simulink model "DFexample"  (R2017a)
settings: Solver=FixedStepAuto  StartTime=0.0  StopTime=600  FixedStep=0.01  RelTol=1e-3
settings Model: Creator=bhannigan  LastModifiedBy=bhannigan

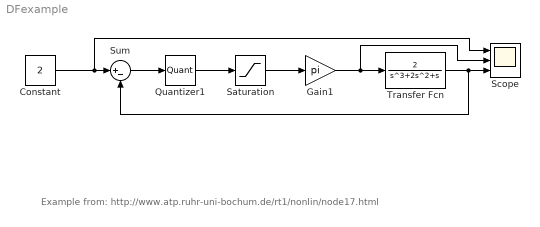
== system DFexample ==
  note: Example from: http://www.atp.ruhr-uni-bochum.de/rt1/nonlin/node17.html
  Constant : Constant  Value=2
  Gain1 : Gain  Gain=pi
  Quantizer1 : Quantizer  QuantizationInterval=2
  Saturation : Saturate  UpperLimit=1  LowerLimit=-1
  Scope : Scope  NumInputPorts=3
  Sum : Sum  Inputs=|+-
  Transfer Fcn : TransferFcn  Numerator=2  Denominator=[1 2 1 0]
  wires:
  Transfer Fcn/1 -> Scope/3, Sum/2
  Constant/1 -> Scope/1, Sum/1
  Saturation/1 -> Gain1/1
  Gain1/1 -> Scope/2, Transfer Fcn/1
  Quantizer1/1 -> Saturation/1
  Sum/1 -> Quantizer1/1
